simulink model "sim_DC_Motor_full_order_model"  (R2024b)
settings: Solver=VariableStepAuto  StartTime=0.0  StopTime=Tsim  RelTol=1e-3
values from neighbouring files (symbols this model uses):
  Ac = [ 0 1 0 ... (first row only)    [DC_Motor_full_order_model.m]    (also in main_SysId_DC_Motor_LS_KF_RO_model.m = [0         1; main_SysId_DC_Motor_LS_RO_model.m = [0         1; main_SysId_DC_Motor_RLS_RO_model.m = [0         1)
  Bc = [0 0 1/l]'    [DC_Motor_full_order_model.m]    (also in main_SysId_DC_Motor_LS_Full_model.m; main_SysId_DC_Motor_LS_KF_RO_model.m = [0; main_SysId_DC_Motor_LS_RO_model.m = [0; main_SysId_DC_Motor_RLS_RO_model.m = [0)
  Ng_i = 0.05    [main_SysId_DC_Motor_LS_Full_model.m]    (also in main_SysId_DC_Motor_LS_KF_RO_model.m = 0.1; main_SysId_DC_Motor_LS_RO_model.m = 0.1; main_SysId_DC_Motor_RLS_RO_model.m = 0.1)
  Ng_theta = 0.05    [main_SysId_DC_Motor_LS_Full_model.m]    (also in main_SysId_DC_Motor_LS_KF_RO_model.m; main_SysId_DC_Motor_LS_RO_model.m; main_SysId_DC_Motor_RLS_RO_model.m)
  Ng_w = 0.1    [main_SysId_DC_Motor_LS_Full_model.m]    (also in main_SysId_DC_Motor_LS_KF_RO_model.m; main_SysId_DC_Motor_LS_RO_model.m; main_SysId_DC_Motor_RLS_RO_model.m = 0.01)
  ts = 1/fs    (= 0.01)    [main_SysId_DC_Motor_LS_Full_model.m]    (also in main_SysId_DC_Motor_LS_KF_RO_model.m = 0.005; main_SysId_DC_Motor_LS_RO_model.m = 0.005; main_SysId_DC_Motor_RLS_RO_model.m = 0.005)
  Vpeak = 2    [main_SysId_DC_Motor_LS_Full_model.m]    (also in main_SysId_DC_Motor_LS_KF_RO_model.m = 5; main_SysId_DC_Motor_LS_RO_model.m = 3; main_SysId_DC_Motor_RLS_RO_model.m = 3)
settings Model: Creator=ricardoaguilera  LastModifiedBy=ricardoaguilera
settings SolverCC: AutoInsertRateTranBlk=on
settings DataIOCC: ReturnWorkspaceOutputs=off

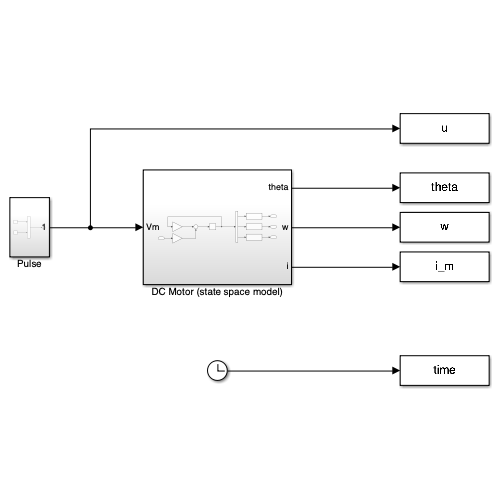
[thumbnail: Simulink's stored preview of the top-level diagram]
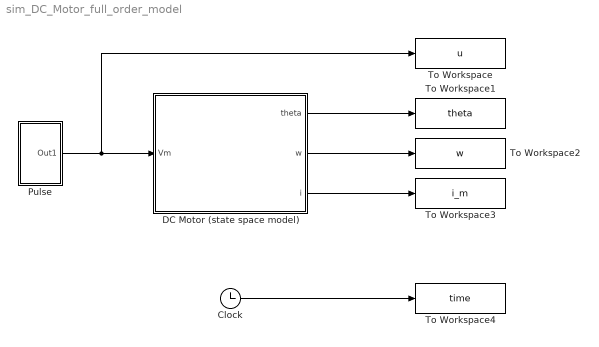
== system sim_DC_Motor_full_order_model ==
  Clock : Clock
  DC Motor (state space model) : Subsystem
  Pulse : Subsystem
  To Workspace : ToWorkspace  VariableName=u  SampleTime=ts
  To Workspace1 : ToWorkspace  VariableName=theta  SampleTime=ts
  To Workspace2 : ToWorkspace  VariableName=w  SampleTime=ts
  To Workspace3 : ToWorkspace  VariableName=i_m  SampleTime=ts
  To Workspace4 : ToWorkspace  VariableName=time  SampleTime=ts
  wires:
  Pulse/1(Out1) -> To Workspace/1, DC Motor (state space model)/1(Vm)
  DC Motor (state space model)/1(theta) -> To Workspace1/1
  DC Motor (state space model)/2(w) -> To Workspace2/1
  DC Motor (state space model)/3(i) -> To Workspace3/1
  Clock/1 -> To Workspace4/1

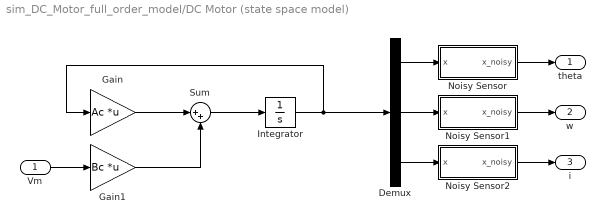
== system sim_DC_Motor_full_order_model/DC Motor (state space model) ==
  Vm : Inport
  Demux : Demux  Outputs=3
  Gain : Gain  Gain=Ac  Multiplication=Matrix(K*u)
  Gain1 : Gain  Gain=Bc  Multiplication=Matrix(K*u)
  Integrator : Integrator
  Noisy Sensor : Subsystem
  Noisy Sensor1 : Subsystem
  Noisy Sensor2 : Subsystem
  Sum : Sum  Inputs=|++
  theta : Outport
  w : Outport  Port=2
  i : Outport  Port=3
  wires:
  Integrator/1 -> Gain/1, Demux/1
  Sum/1 -> Integrator/1
  Vm/1 -> Gain1/1
  Gain1/1 -> Sum/2
  Gain/1 -> Sum/1
  Noisy Sensor/1(x_noisy) -> theta/1
  Demux/1 -> Noisy Sensor/1(x)
  Demux/2 -> Noisy Sensor1/1(x)
  Demux/3 -> Noisy Sensor2/1(x)
  Noisy Sensor1/1(x_noisy) -> w/1
  Noisy Sensor2/1(x_noisy) -> i/1

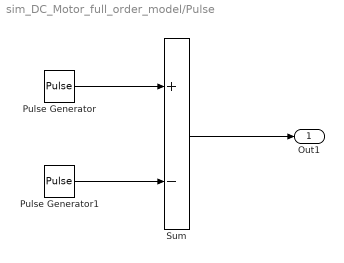
== system sim_DC_Motor_full_order_model/Pulse ==
  Pulse Generator : DiscretePulseGenerator  PulseType=Time based  Amplitude=Vpeak  Period=10  PulseWidth=10  PhaseDelay=2
  Pulse Generator1 : DiscretePulseGenerator  PulseType=Time based  Amplitude=Vpeak  Period=10  PulseWidth=10  PhaseDelay=6
  Sum : Sum  Inputs=+-
  Out1 : Outport
  wires:
  Sum/1 -> Out1/1
  Pulse Generator/1 -> Sum/1
  Pulse Generator1/1 -> Sum/2

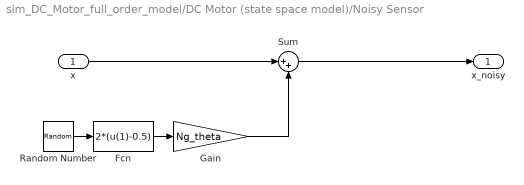
== system sim_DC_Motor_full_order_model/DC Motor (state space model)/Noisy Sensor ==
  x : Inport
  Fcn : Fcn  Expr=2*(u(1)-0.5)
  Gain : Gain  Gain=Ng_theta
  Random Number : RandomNumber  SampleTime=ts
  Sum : Sum  Inputs=|++
  x_noisy : Outport
  wires:
  Sum/1 -> x_noisy/1
  Gain/1 -> Sum/2
  Fcn/1 -> Gain/1
  x/1 -> Sum/1
  Random Number/1 -> Fcn/1

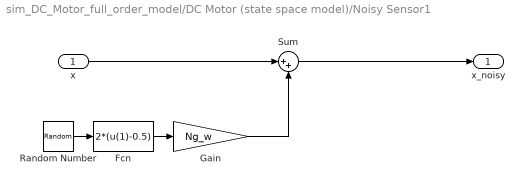
== system sim_DC_Motor_full_order_model/DC Motor (state space model)/Noisy Sensor1 ==
  x : Inport
  Fcn : Fcn  Expr=2*(u(1)-0.5)
  Gain : Gain  Gain=Ng_w
  Random Number : RandomNumber  SampleTime=ts
  Sum : Sum  Inputs=|++
  x_noisy : Outport
  wires:
  Sum/1 -> x_noisy/1
  Gain/1 -> Sum/2
  Fcn/1 -> Gain/1
  x/1 -> Sum/1
  Random Number/1 -> Fcn/1

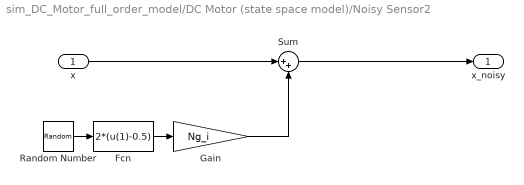
== system sim_DC_Motor_full_order_model/DC Motor (state space model)/Noisy Sensor2 ==
  x : Inport
  Fcn : Fcn  Expr=2*(u(1)-0.5)
  Gain : Gain  Gain=Ng_i
  Random Number : RandomNumber  SampleTime=ts
  Sum : Sum  Inputs=|++
  x_noisy : Outport
  wires:
  Sum/1 -> x_noisy/1
  Gain/1 -> Sum/2
  Fcn/1 -> Gain/1
  x/1 -> Sum/1
  Random Number/1 -> Fcn/1
